simulink model "carestimation_model"  (Simulink 7.9)
settings: Solver=ode45  StartTime=0.0  StopTime=10.0  RelTol=1e-3
settings Model: Creator=doris_yingxin  LastModifiedBy=doris_yingxin

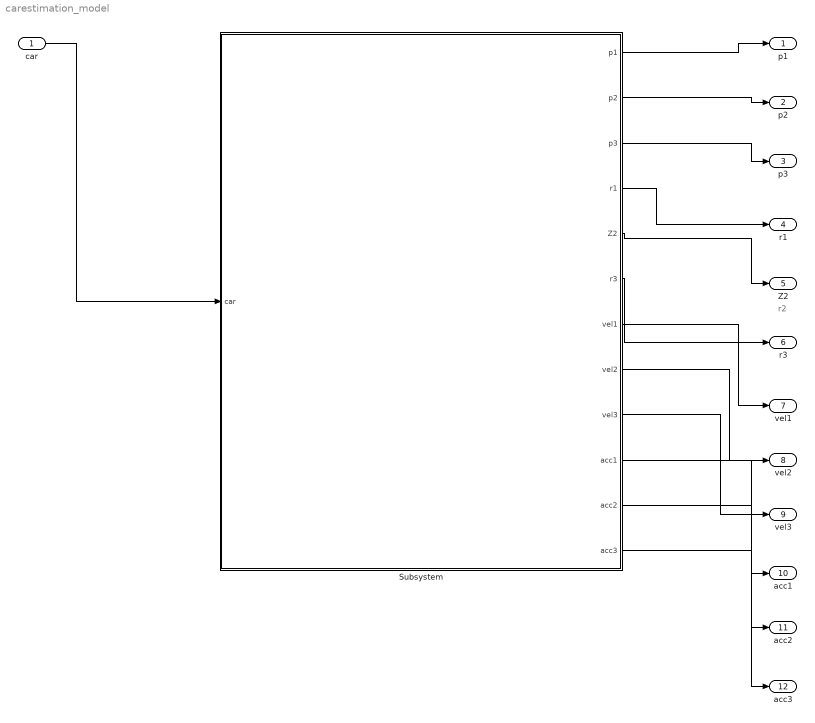
== system carestimation_model ==
  note: r2
  car : Inport
  Subsystem : Subsystem
  p1 : Outport
  p2 : Outport  Port=2
  p3 : Outport  Port=3
  r1 : Outport  Port=4
  Z2 : Outport  Port=5
  r3 : Outport  Port=6
  vel1 : Outport  Port=7
  vel2 : Outport  Port=8
  vel3 : Outport  Port=9
  acc1 : Outport  Port=10
  acc2 : Outport  Port=11
  acc3 : Outport  Port=12
  wires:
  car/1 -> Subsystem/1(car)
  Subsystem/1(p1) -> p1/1
  Subsystem/2(p2) -> p2/1
  Subsystem/3(p3) -> p3/1
  Subsystem/4(r1) -> r1/1
  Subsystem/5(Z2) -> Z2/1
  Subsystem/6(r3) -> r3/1
  Subsystem/7(vel1) -> vel1/1
  Subsystem/8(vel2) -> vel2/1
  Subsystem/9(vel3) -> vel3/1
  Subsystem/10(acc1) -> acc1/1
  Subsystem/11(acc2) -> acc2/1
  Subsystem/12(acc3) -> acc3/1

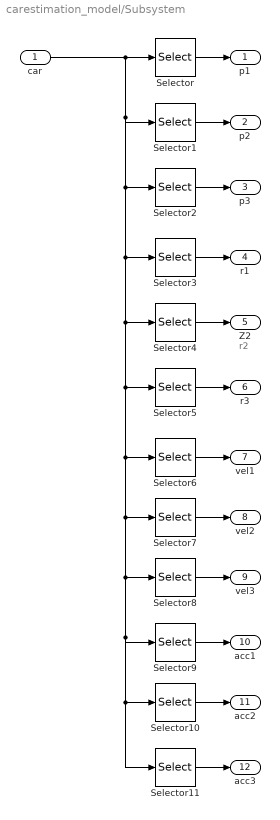
== system carestimation_model/Subsystem ==
  note: r2
  car : Inport
  Selector : Selector  NumberOfDimensions=12  InputPortWidth=3  IndexOptions=Index vector (dialog),Index vector (dialog),Index vector (dialog),Index vector (dialog),Index vector (dialog),Index vector (dialog),Index vector (dialog),Index vector (dialog),Index vector (dialog),Index vector (dialog),Index vector (dialog),Index vector (dialog)  Indices=1,1,1,1,1,1,1,1,1,1,1,1  OutputSizes=1,1,1,1,1,1,1,1,1,1,1,1
  Selector1 : Selector  NumberOfDimensions=12  InputPortWidth=3  IndexOptions=Index vector (dialog),Index vector (dialog),Index vector (dialog),Index vector (dialog),Index vector (dialog),Index vector (dialog),Index vector (dialog),Index vector (dialog),Index vector (dialog),Index vector (dialog),Index vector (dialog),Index vector (dialog)  Indices=1,1,2,1,1,1,1,1,1,1,1,1  OutputSizes=1,1,1,1,1,1,1,1,1,1,1,1
  Selector{2..11} (10 alike) : Selector  NumberOfDimensions=12  InputPortWidth=3  IndexOptions=Index vector (dialog),Index vector (dialog),Index vector (dialog),Index vector (dialog),Index vector (dialog),Index vector (dialog),Index vector (dialog),Index vector (dialog),Index vector (dialog),Index vector (dialog),Index vector (dialog),Index vector (dialog)  Indices=1,1,3,1,1,1,1,1,1,1,1,1  OutputSizes=1,1,1,1,1,1,1,1,1,1,1,1
  p1 : Outport
  p2 : Outport  Port=2
  p3 : Outport  Port=3
  r1 : Outport  Port=4
  Z2 : Outport  Port=5
  r3 : Outport  Port=6
  vel1 : Outport  Port=7
  vel2 : Outport  Port=8
  vel3 : Outport  Port=9
  acc1 : Outport  Port=10
  acc2 : Outport  Port=11
  acc3 : Outport  Port=12
  wires:
  Selector/1 -> p1/1
  Selector1/1 -> p2/1
  Selector2/1 -> p3/1
  Selector3/1 -> r1/1
  Selector4/1 -> Z2/1
  Selector5/1 -> r3/1
  Selector6/1 -> vel1/1
  Selector7/1 -> vel2/1
  Selector8/1 -> vel3/1
  Selector9/1 -> acc1/1
  Selector10/1 -> acc2/1
  Selector11/1 -> acc3/1
  car/1 -> Selector/1, Selector1/1, Selector2/1, Selector3/1, Selector4/1, Selector5/1, Selector6/1, Selector7/1, Selector8/1, Selector9/1, Selector10/1, Selector11/1
